simulink subsystem "Main_Kalman_1D"  (R2024a)
settings: Solver=VariableStepAuto  StartTime=0.0  StopTime=10.0  RelTol=1e-3
undefined symbols (not defined in the file): A_pend, B_pend, Q_kf, R_kf
settings Model: Creator=Peter  LastModifiedBy=Peter

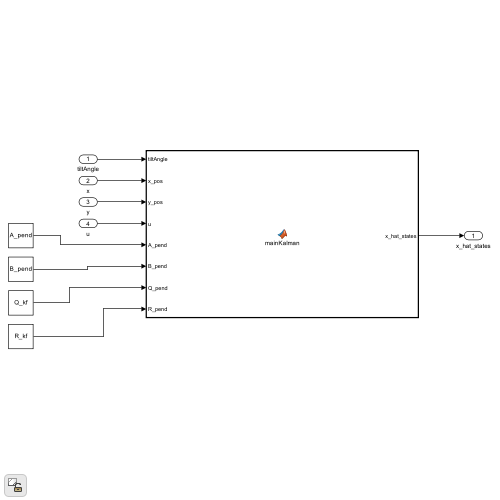
[thumbnail: Simulink's stored preview of the top-level diagram]
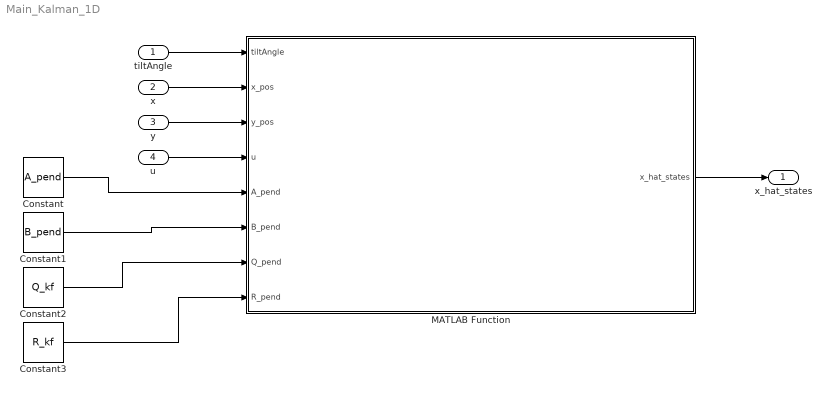
== system Main_Kalman_1D ==
  tiltAngle : Inport  OutDataTypeStr=single
  x : Inport  Port=2  OutDataTypeStr=single
  y : Inport  Port=3  OutDataTypeStr=single
  u : Inport  Port=4  OutDataTypeStr=single
  Constant : Constant  Value=A_pend
  Constant1 : Constant  Value=B_pend
  Constant2 : Constant  Value=Q_kf
  Constant3 : Constant  Value=R_kf
  MATLAB Function : MATLAB Function  TreatAsAtomicUnit=on
  x_hat_states : Outport  OutDataTypeStr=single
  wires:
  MATLAB Function/1(x_hat_states) -> x_hat_states/1
  x/1 -> MATLAB Function/2(x_pos)
  tiltAngle/1 -> MATLAB Function/1(tiltAngle)
  y/1 -> MATLAB Function/3(y_pos)
  u/1 -> MATLAB Function/4(u)
  Constant/1 -> MATLAB Function/5(A_pend)
  Constant1/1 -> MATLAB Function/6(B_pend)
  Constant2/1 -> MATLAB Function/7(Q_pend)
  Constant3/1 -> MATLAB Function/8(R_pend)

== matlab function Main_Kalman_1D/MATLAB Function ==
  data: tiltAngle input single; x_hat_states output single; x_pos input single; y_pos input single; u input; A_pend input; B_pend input; Q_pend input; R_pend input
function x_hat_states = mainKalman(tiltAngle,x_pos,y_pos,u, A_pend, B_pend, Q_pend, R_pend)
% kalman_filter  Discrete-time Kalman filter for 2-wheeled self-balancing robot
% States: x = [ x; x_dot; theta; theta_dot ]  (4x1)
% Measurements assumed y = [ x_encoder; theta_accel; theta_dot_gyro ] (3x1)
%
% Inputs:
%   y   (3x1)   measurement vector
%   u   (1x1)   control input
%   A   (4x4)   state transition matrix (discrete)
%   B   (4x1)   input matrix
%   Q   (4x4)   process noise covariance
%   R   (3x3)   measurement noise covariance
%   x0  (4x1)   initial state (used on reset)
%   P0  (4x4)   initial covariance (used on reset)
%   reset (scalar logical/int)  set to 1 to reinitialize x_hat := x0, P := P0
%
% Outputs:
%   x_hat (4x1)  filtered state estimate
%   P_out (4x4)  current covariance
%
% NOTE: This code uses single precision to be suitable for embedded targets.

    A = single(A_pend);
    B = single(B_pend);
    Q = single(Q_pend);
    R = single(R_pend);
    y = single([tiltAngle;x_pos]);

    % Voltage to force conversion in motor steady state
    params.N = 42;
    params.Kt = 0.005671;
    params.eta = 0.9;
    params.Ke = 0.3; 
    params.R = 3.428571;
    params.useBackEmf = false;
    params.r = 0.03;
    F = V_to_force(u, 0, params);

    u = single(F);
    
    % Dimensions (hard-coded to avoid dynamic size issues)
    nx = 4;   % state dimension
    nz = 2;   % measurement dimension (y size)
    
    persistent xhat P initialized

    if isempty(initialized)
        xhat = zeros(nx,1,'single');
        P    = eye(nx,'single') * single(1e-3);
        initialized = true;
    end
    
        H = single([ 1 0 0 0;    % x_encoder measures x
                     0 0 1 0]);   % theta
        
        % Prediction step
        x_pred = A * xhat + B * u;           % 4x1
        P_pred = A * P * A' + Q;             % 4x4
        
        % Update step
        y_pred = H * x_pred;                  % 2x1
        innov = y - y_pred;                   % 2x1
        
        % Innovation covariance S = H*P_pred*H' + R  (2x2)
        S = H * P_pred * H' + R;
        
        % Kalman gain K = P_pred * H' * inv(S)  (4x2)
        S_inv = inv(S);                       % 2x2
        K = P_pred * H' * S_inv;              % 4x2
        
        % State update
        xhat = x_pred + K * innov;            % 4x1
        
        % Joseph stabilized covariance update:
        I = eye(nx,'single');
        P = (I - K*H) * P_pred * (I - K*H)' + K * R * K';
        
        % Outputs
        x_hat_states = xhat;
        %P_out = P;
    
end

function F = V_to_force(V, omega_w, params)
% V_to_force  Convert applied voltage (V) to wheel force (N) - steady-state approx
%   V         : applied motor voltage (scalar) [V]
%   omega_w   : wheel angular speed (rad/s) (scalar)
%   params    : struct with fields
%       R    - motor resistance (ohm)
%       Kt   - torque constant (N*m/A)
%       Ke   - back-emf constant (V/(rad/s))
%       N    - gearbox ratio (omega_motor / omega_wheel)
%       r    - wheel radius (m)
%       eta  - drivetrain efficiency (0..1) (default 1)
%       useBackEmf - boolean (default true)
%
% Output:
%   F : force at wheel (N)

if ~isfield(params,'eta'), params.eta = 1; end
if ~isfield(params,'useBackEmf'), params.useBackEmf = true; end

R  = params.R;
Kt = params.Kt;
Ke = params.Ke;
N  = params.N;
r  = params.r;
eta = params.eta;

% linear gain (N/V)
alpha = (eta * N * Kt) / (r * R);

if params.useBackEmf
    % back-emf term (depends on wheel speed)
    beta = - (eta * N^2 * Kt * Ke) / (r * R);
    F = alpha * V + beta * omega_w;
else
    F = alpha * V;
end

end
